simulink model "project8_week1"  (R2020b)
settings: Solver=VariableStepAuto  StartTime=0.0  StopTime=10.0  RelTol=1e-3
settings Model: Creator=RASIKA MALGI  LastModifiedBy=RASIKA MALGI

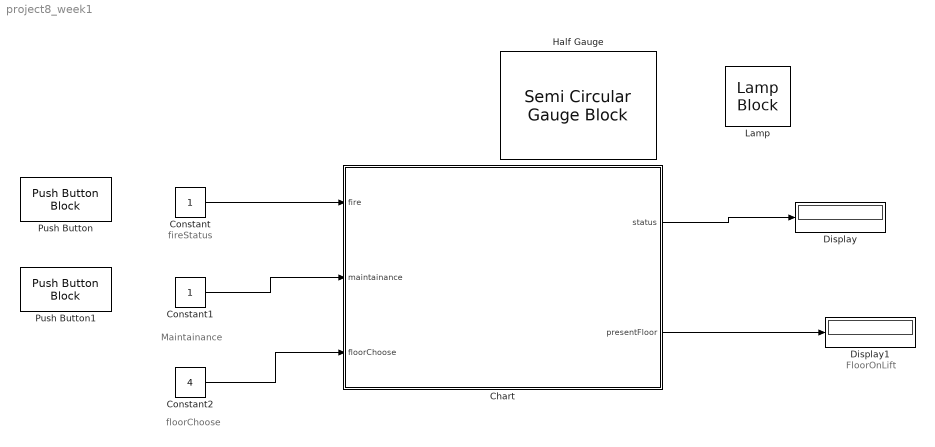
== system project8_week1 ==
  note: floorChoose
  note: FloorOnLift
  note: Maintainance
  note: fireStatus
  Chart : Stateflow chart  TreatAsAtomicUnit=on
  Constant : Constant
  Constant1 : Constant
  Constant2 : Constant  Value=4
  Display : Display
  Display1 : Display
  Half Gauge : SemiCircularGaugeBlock  ScaleMax=5  TickInterval=1
  Lamp : LampBlock
  Push Button : PushButtonBlock
  Push Button1 : PushButtonBlock
  wires:
  Chart/2(presentFloor) -> Display1/1
  Chart/1(status) -> Display/1
  Constant/1 -> Chart/1(fire)
  Constant1/1 -> Chart/2(maintainance)
  Constant2/1 -> Chart/3(floorChoose)

== stateflow chart project8_week1/Chart ==
  state LiftOperation [parallel]
    entry:
    status=0;
    settings: executionOrder=1
    state LiftOn
      (history)
      state groundFloor
        entry:
        status=1;
        during:
        presentFloor=0;
        FloorCheck(presentFloor);
        exit:
        status=0;
      state firstFloor
        entry:
        status=1;
        during:
        presentFloor=1;
        FloorCheck(presentFloor);
        exit:
        status=0;
      state secondFloor
        entry:
        status=1;
        during:
        presentFloor=2;
        FloorCheck(presentFloor);
        exit:
        status=0;
        after(1,sec);
      state thirdFloor
        entry:
        status=1;
        during:
        presentFloor=3;
        FloorCheck(presentFloor);
        exit:
        status=0;
        after(1,sec);
      state fourthFloor
        entry:
        status=1
        during:
        presentFloor=4;
        FloorCheck(presentFloor);
        exit:
        status=0;
      state fifthFloor
        entry:
        status=1;
        during:
        presentFloor=5;
        FloorCheck(presentFloor);
        exit:
        status=0;
      (default) -> groundFloor
      groundFloor -> firstFloor : up
      firstFloor -> groundFloor [order 2] : down
      firstFloor -> secondFloor [order 1] : up
      secondFloor -> firstFloor [order 2] : down
      secondFloor -> thirdFloor [order 1] : up
      thirdFloor -> secondFloor [order 2] : down
      thirdFloor -> fourthFloor [order 1] : up
      fourthFloor -> thirdFloor [order 1] : down
      fourthFloor -> fifthFloor [order 2] : up
      fifthFloor -> fourthFloor : down
    state LiftOff
      entry:
      status=0;
    (default) -> LiftOn
    LiftOn -> LiftOff : [fire==1||maintainance==1]
    LiftOff -> LiftOn : [fire==0||maintainance==0]
  state Alarm [parallel]
    settings: executionOrder=2
    (default) -> (junction 25) : % Alarm Loop
        | {alarmLevel=fire;}
    (junction 25) -> (junction 29)
    (junction 26) -> (junction 35) [order 2] : [alarmLevel==1]{send(off);}
    (junction 29) -> (junction 26) [order 1] : [1]
    (junction 27) -> (junction 29)
    (junction 26) -> (junction 27) [order 1] : [alarmLevel==0]{send(on);}
    (junction 35) -> (junction 28)
    (junction 29) -> (junction 30) [order 2]
    (junction 28) -> (junction 27)
  state y = FloorCheck(Floor) [function]
    (default) -> (junction 45)
    (junction 45) -> (junction 44) [order 3] : [floorChoose<Floor]{
        | send(down);
        | disp('LiftMovingDown');}
    (junction 45) -> (junction 46) [order 1] : [floorChoose>Floor]{
        | send(up);
        | disp('LiftMovingUp');}
    (junction 44) -> (junction 47)
    (junction 45) -> (junction 48) [order 2] : [floorChoose==Floor]{
        | disp('CurrentFloor');}
    (junction 46) -> (junction 49)
    (junction 47) -> (junction 48)
    (junction 49) -> (junction 48)
    (junction 48) -> (junction 50)
  data: Floor function_input; y function_output; status output; fire input; maintainance input; presentFloor output; alarmLevel local; floorChoose input
  events: on local FUNCTION_CALL_EVENT; off local FUNCTION_CALL_EVENT; up local FUNCTION_CALL_EVENT; down local FUNCTION_CALL_EVENT
